simulink model "arduino_serial_sendreceive"  (R2023b)
settings: Solver=FixedStepAuto  StartTime=0.0  StopTime=inf  RelTol=1e-3  EnableMultiTasking=on
libraries: arduinolib x3, realtime_examples_misc x2, simulink x1
settings Model: SimulationMode=external  ExtModeTrigDuration=2  Creator=The MathWorks, Inc.  LastModifiedBy=maxju
settings SolverCC: AlgebraicLoopSolver=TrustRegion
settings DataIOCC: ReturnWorkspaceOutputs=off
settings OptimizationCC: PassReuseOutputArgsThreshold=0  MaxStackSize=64
settings DebuggingCC: ParameterTunabilityLossMsg=error  UnconnectedInputMsg=warning  UnconnectedOutputMsg=warning  UnconnectedLineMsg=warning  ArithmeticOperatorsInVariantConditions=warning
settings HardwareCC: ProdBitPerInt=16  ProdBitPerPointer=16  ProdBitPerSizeT=16  ProdBitPerPtrDiffT=16  ProdLargestAtomicFloat=None  ProdWordSize=8  ProdHWDeviceType=Atmel->AVR  UseEmbeddedCoderFeatures=off  UseSimulinkCoderFeatures=off
settings ModelReferenceCC: EnableRefExpFcnMdlSchedulingChecks=on
settings SFSimCC: SimUseLocalCustomCode=off  MATLABDynamicMemAlloc=off
settings RTWCC: Description=Embedded Coder  SystemTargetFile=ert.tlc  HardwareBoard=Arduino Mega 2560  TemplateMakefile=ert_default_tmf  GenerateReport=on  RTWUseLocalCustomCode=off  Toolchain=Arduino AVR  BuildConfiguration=Faster Runs  LaunchReport=on  DLArmComputeVersion=19.05
settings CodeAppCC: ForceParamTrailComments=on  OperatorAnnotations=on
settings ERTTargetCC: ERTCustomFileBanners=off  SupportContinuousTime=on  SupportNonInlinedSFcns=on  RemoveResetFunc=off  SupportVariableSizeSignals=on  ModelStepFunctionPrototypeControlCompliant=off

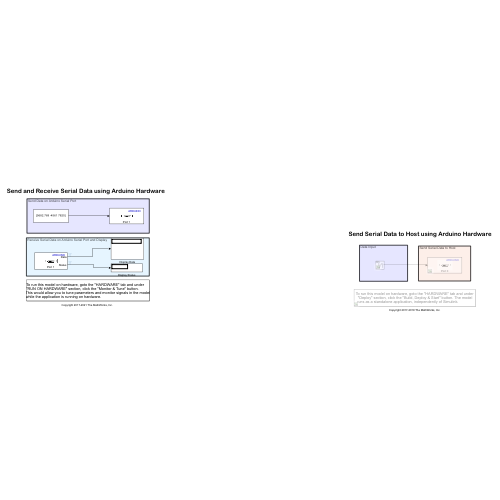
[thumbnail: Simulink's stored preview of the top-level diagram]
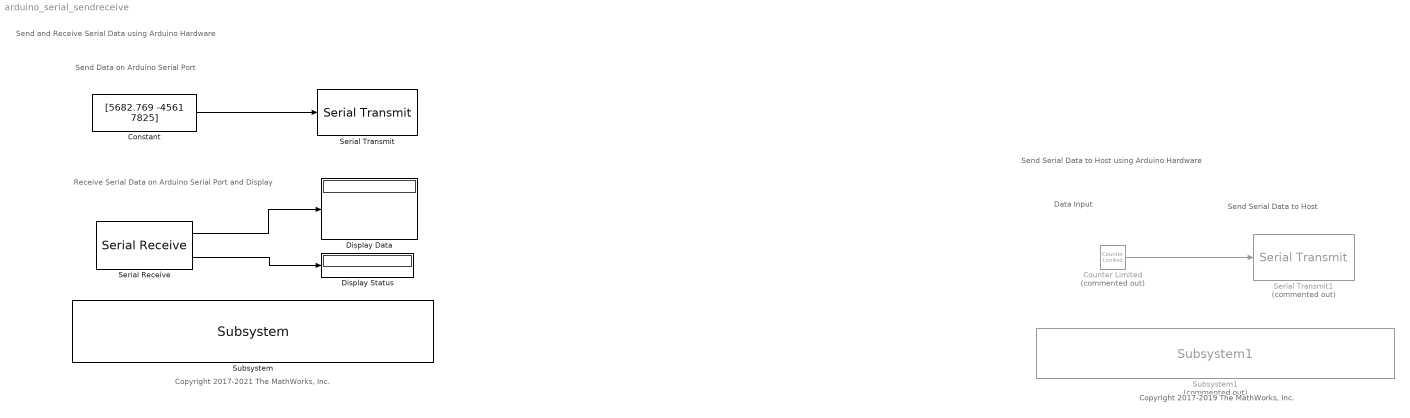
== system arduino_serial_sendreceive ==
  note: Receive Serial Data on Arduino Serial Port and Display
  note: Send Data on Arduino Serial Port
  note: Send and Receive Serial Data using Arduino Hardware
  note: Copyright 2017-2021 The MathWorks, Inc.
  note: Send Serial Data to Host using Arduino Hardware
  note: Send Serial Data to Host
  note: Data Input
  note: Copyright 2017-2019 The MathWorks, Inc.
  Constant : Constant  Value=[5682.769 -4561 7825]  OutDataTypeStr=double  SampleTime=0.1
  Counter Limited : simulink/Sources/Counter Limited  Commented=on  uplimit=7  tsamp=1
  Display Data : Display
  Display Status : Display
  Serial Receive : arduinolib/Serial Receive  isARMArch=off  portNumber=1  DataType=double  Datalength=3  SampleTime=0.1  showOutStatus=on  blockPlatform=arduino
  Serial Transmit : arduinolib/Serial Transmit  portNumber=1  sendmode=write  label=GPS_latitude  sendformat=Decimal  floatprecision=5  blockPlatform=arduino
  Serial Transmit1 : arduinolib/Serial Transmit  Commented=on  portNumber=0  sendmode=println  label=Counter_val :  sendformat=Decimal  floatprecision=2  blockPlatform=arduino
  Subsystem : realtime_examples_misc/Subsystem  SystemSampleTime=-1  VariantActivationTime=update diagram  AllowFlexibleInterface=on  Latency=0  AutoFrameSizeCalculation=off
  Subsystem1 : realtime_examples_misc/Subsystem1  Commented=on  SystemSampleTime=-1  VariantActivationTime=update diagram  AllowFlexibleInterface=on  Latency=0  AutoFrameSizeCalculation=off
  wires:
  Constant/1 -> Serial Transmit/1
  Serial Receive/1 -> Display Data/1
  Serial Receive/2 -> Display Status/1
  Counter Limited/1 -> Serial Transmit1/1
